simulink model "wind_turbine"  (R2020a)
settings: Solver=VariableStepAuto  StartTime=0.0  StopTime=1  RelTol=1e-3
libraries: powerlib x5, re_lib x1
settings Model: Creator=sameeraa  LastModifiedBy=sameeraa

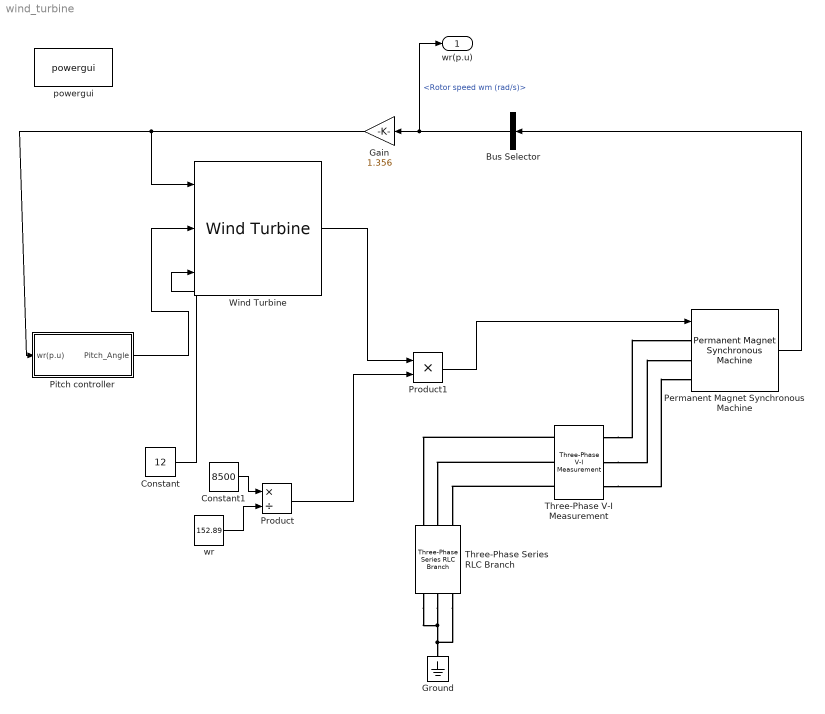
== system wind_turbine ==
  Bus Selector : BusSelector  OutputSignals=Rotor speed wm (rad/s)
  Constant : Constant  Value=12
  Constant1 : Constant  Value=8500
  Gain : Gain  Gain=1.356
  Ground : powerlib/Elements/Ground  LConnTagsString=a
  Permanent Magnet Synchronous Machine : powerlib/Machines/Permanent Magnet Synchronous Machine  NbPhases=3  FluxDistribution=Sinusoidal  RotorType=Round  MechanicalLoad=Torque Tm  PresetModel=No  ShowDetailedParameters=on  MeasurementBus=off  Resistance=0.0485  Inductance=8.5e-3  dqInductances=[8.5e-3,8.5e-3]  La=0.000395  MachineConstant=Flux linkage established by magnets (V.s)  Flux=0.1194  VoltageCst=86.6271  TorqueCst=0.7164  Flat=120  Mechanical=[0.0027 0.0004924 4 0]  PolePairs=4  InitialConditions=[0,0, 0,0]  InitialConditions5ph=[0 0 0 0 0 0]  RefAngle=90 degrees behind phase A axis (modified Park)  IterativeDiscreteModel=Trapezoidal non iterative  TsBlock=-1  TsPowergui=0
  Pitch controller : Subsystem
  Product : Product  Inputs=*/
  Product1 : Product
  Three-Phase Series RLC Branch : powerlib/Elements/Three-Phase Series RLC Branch  LConnTagsString=A|B|C  RConnTagsString=A|B|C  BranchType=R  Resistance=1  Inductance=1e-3  Capacitance=1e-6  Measurements=None
  Three-Phase V-I Measurement : powerlib/Measurements/Three-Phase V-I Measurement  VoltageMeasurement=no  SetLabelV=off  LabelV=Vabc  Vpu=off  VpuLL=off  CurrentMeasurement=no  SetLabelI=off  LabelI=Iabc  Ipu=off  Pbase=100e6  Vbase=500e3  OutputType=Complex  PhasorSimulation=off  PSBequivalent=0
  Wind Turbine : re_lib/Wind Generation/Wind Turbine  Pnom=8.5e3  Pelec_base=8.5e3/0.9  wind_base=12  P_wind_base=0.8  speed_nom=1  pitch_angle=0  c1_c6="[0.51763          116          0.4            5           21     0.006795]"  cp_nom=0.48  lambda_nom=8.1
      settings: SourceProductBaseCode=PS
  powergui : powerlib/powergui  Priority=1  SimulationMode=Discrete  SampleTime=5e-6  frequency=60  Iterations=50  frequencyindice=0  Pbase=100e6  ErrMax=1e-4  UnitsV=kV  UnitsW=MW  buscounter=0  FunctionMessages=off  echomessages=off  EnableUseOfTLC=off  CurrentSourceSwitches=off  DisableSnubberDevices=off  DisableRonSwitches=off  DisableVfSwitches=off  DisplayEquations=off  AutomaticDiscreteSolvers=off  SolverType=Tustin/Backward Euler (TBE)  Interpol=off  ExternalGateDelay=off  methode=off  Ts=100  x0status=blocks  SPID=on  SwTol=0  HookPort=off  NonlinearTolerance=1e-4  nMaxIteration=100  ContinueOnMaxIteration=off  RestoreLinks=warning  ResistiveCurrentMeasurement=off  Frange=[0:2:500]  Ylog=off  Xlog=on  ShowGrid=off  save=off  variable=ZData  structure=0  ZoomFFT=off  StartTime=0.0  cycles=1  DisplayStyle=1  fundamental=60  FreqAxis=off  MaxFrequency=1000  frequencyindicesteady=1  RmsSteady=1  display=off
  wr : Constant  Value=152.89
  wr(p.u) : Outport
  wires:
  Pitch controller/1(Pitch_Angle) -> Wind Turbine/2
  Constant/1 -> Wind Turbine/3
  Product/1 -> Product1/2
  wr/1 -> Product/2
  Constant1/1 -> Product/1
  Product1/1 -> Permanent Magnet Synchronous Machine/1
  Permanent Magnet Synchronous Machine/1 -> Bus Selector/1
  Bus Selector/1 -> wr(p.u)/1, Gain/1  "<Rotor speed wm (rad/s)>"
  Gain/1 -> Wind Turbine/1, Pitch controller/1(wr(p.u))
  Wind Turbine/1 -> Product1/1
  connections:
  Three-Phase V-I Measurement/LConn1 -- Permanent Magnet Synchronous Machine/LConn1
  Three-Phase V-I Measurement/LConn2 -- Permanent Magnet Synchronous Machine/LConn2
  Three-Phase V-I Measurement/LConn3 -- Permanent Magnet Synchronous Machine/LConn3
  Three-Phase V-I Measurement/RConn1 -- Three-Phase Series RLC Branch/LConn1
  Three-Phase V-I Measurement/RConn2 -- Three-Phase Series RLC Branch/LConn2
  Three-Phase V-I Measurement/RConn3 -- Three-Phase Series RLC Branch/LConn3
  Three-Phase Series RLC Branch/RConn1 -- Three-Phase Series RLC Branch/RConn3 -- Ground/LConn1 -- Three-Phase Series RLC Branch/RConn2

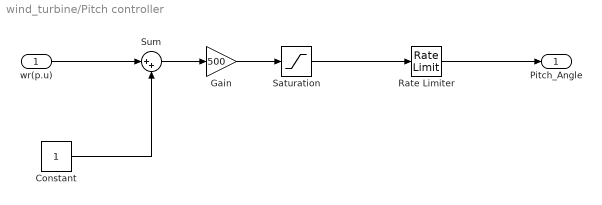
== system wind_turbine/Pitch controller ==
  wr(p.u) : Inport
  Constant : Constant
  Gain : Gain  Gain=500
  Rate Limiter : RateLimiter  RisingSlewLimit=2  FallingSlewLimit=-2  SampleTimeMode=inherited
  Saturation : Saturate  UpperLimit=45  LowerLimit=0
  Sum : Sum  Inputs=|++
  Pitch_Angle : Outport
  wires:
  wr(p.u)/1 -> Sum/1
  Constant/1 -> Sum/2
  Sum/1 -> Gain/1
  Gain/1 -> Saturation/1
  Saturation/1 -> Rate Limiter/1
  Rate Limiter/1 -> Pitch_Angle/1
